simulink model "dcdctest"  (R2023b)
settings: Solver=VariableStepAuto  StartTime=0.0  StopTime=10  RelTol=1e-3
values from neighbouring files (symbols this model uses):
  cell_cap_Ah = 2.2    [find_maximum_ovlp.m]    (also in main.m)
  dst_q_cls = zeros(50, 2)    [main.m]
  dst_trg_soc_av = zeros(50, 1)    [main.m]
  soc = soc_in    [balance_costF.m]    (also in find_maximum_ovlp.m = fix(rand (1, cell_count) * 100); log_clustering.m; main.m = [39    39    20    72    81    92    51    11    60]; plot_final.m)
  src_q_cls = zeros(50, 2)    [main.m]
  src_trg_soc_av = zeros(50, 1)    [main.m]
undefined symbols (not defined in the file or in its folder): Ion, Lithium
libraries: spsIdealSwitchLib x18, spsBatteryLib x12, spsControlledCurrentSourceLib x8, spsVoltageMeasurementLib x8, simulink x4, slpidlib x3, spspowerguiLib x2
(part 1 of 2)
settings Model: NumberOfSteps=100  Creator=10661025  LastModifiedBy=10661025

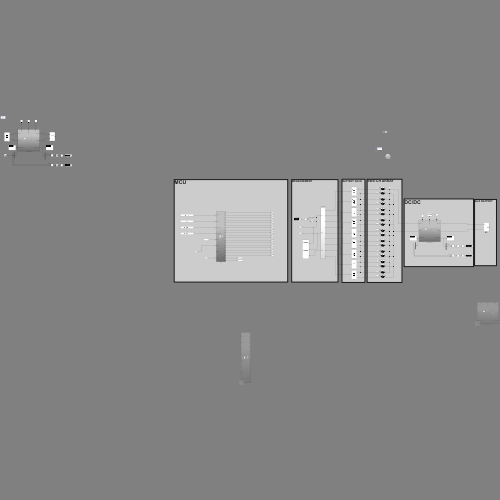
[thumbnail: Simulink's stored preview of the top-level diagram]
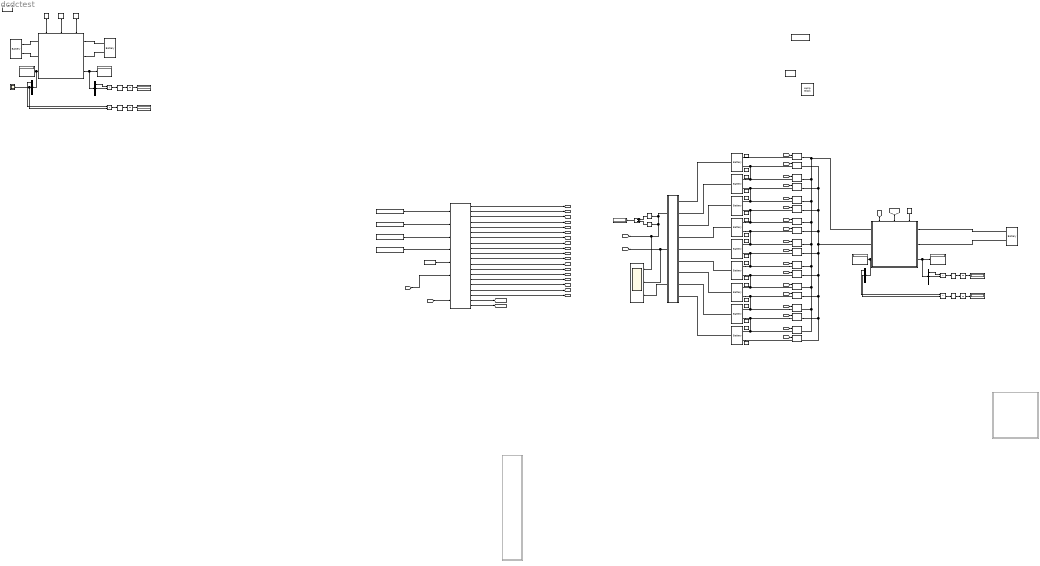
== system dcdctest ==
  note: MCU
  note: DC/DC
  note: MEASUREMENT
  note: BATTERY PACK
  note: SWITCH ARRAY
  note: neg
  note: pos
  note: AUX BATTERY
  Abs{,1..3} (4 alike) : Abs  SaturateOnIntegerOverflow=off
  B1 : spsBatteryLib/Battery  BatType=Lithium-Ion  ShowTempParam=off  ThermalPreset=no  ShowAgeParam=off  NomV=50  NomQ=2.2  SOC=soc(1, 1)  Batt_Tr=30  PresetModel=on  MaxQ=2.2  MinV=37.5  FullV=58.1994  Dis_rate=0.95652  R=0.22727  Normal_OP=1.9896  expZone="[54.0193     0.108087]"  current=[6.5 13 32.5]  Units=Time  Tci=20  NomT=20  T2=-30  MaxQ2=4.8  FullV2=7.1  Normal_OP2=5.655  expZone2="[6.58           1]"  Rca=0.6  ti=2000  Dp=0  Neq0=0  Tsim=1e6  Ta1=25  Qeol=5.4*0.9  Reol=0.013333*1.2  Char_age=[2.3478, 3]  Dis_age=[2.3478, 10]  N1=1500  N2=10500  N3=1000  N4=1400  Ta2=45  N5=950
  B10 : spsBatteryLib/Battery  BatType=Lithium-Ion  ShowTempParam=off  ThermalPreset=no  ShowAgeParam=off  NomV=12  NomQ=60  SOC=soc(1, 1)  Batt_Tr=30  PresetModel=on  MaxQ=60  MinV=9  FullV=13.9678  Dis_rate=26.087  R=0.002  Normal_OP=54.2609  expZone="[12.9646      2.94783]"  current=[6.5 13 32.5]  Units=Time  Tci=20  NomT=20  T2=-30  MaxQ2=4.8  FullV2=7.1  Normal_OP2=5.655  expZone2="[6.58           1]"  Rca=0.6  ti=2000  Dp=0  Neq0=0  Tsim=1e6  Ta1=25  Qeol=5.4*0.9  Reol=0.013333*1.2  Char_age=[2.3478, 3]  Dis_age=[2.3478, 10]  N1=1500  N2=10500  N3=1000  N4=1400  Ta2=45  N5=950
  B11 : spsBatteryLib/Battery  BatType=Lithium-Ion  ShowTempParam=off  ThermalPreset=no  ShowAgeParam=off  NomV=3.7  NomQ=2.2  SOC=soc(1, 8)  Batt_Tr=30  PresetModel=on  MaxQ=2.2  MinV=2.775  FullV=4.3068  Dis_rate=0.95652  R=0.016818  Normal_OP=1.9896  expZone="[3.9974     0.10809]"  current=[6.5 13 32.5]  Units=Time  Tci=20  NomT=20  T2=-30  MaxQ2=4.8  FullV2=7.1  Normal_OP2=5.655  expZone2="[6.58           1]"  Rca=0.6  ti=2000  Dp=0  Neq0=0  Tsim=1e6  Ta1=25  Qeol=5.4*0.9  Reol=0.013333*1.2  Char_age=[2.3478, 3]  Dis_age=[2.3478, 10]  N1=1500  N2=10500  N3=1000  N4=1400  Ta2=45  N5=950
  B12 : spsBatteryLib/Battery  BatType=Lithium-Ion  ShowTempParam=off  ThermalPreset=no  ShowAgeParam=off  NomV=3.7  NomQ=2.2  SOC=soc(1, 9)  Batt_Tr=30  PresetModel=on  MaxQ=2.2  MinV=2.775  FullV=4.3068  Dis_rate=0.95652  R=0.016818  Normal_OP=1.9896  expZone="[3.9974     0.10809]"  current=[6.5 13 32.5]  Units=Time  Tci=20  NomT=20  T2=-30  MaxQ2=4.8  FullV2=7.1  Normal_OP2=5.655  expZone2="[6.58           1]"  Rca=0.6  ti=2000  Dp=0  Neq0=0  Tsim=1e6  Ta1=25  Qeol=5.4*0.9  Reol=0.013333*1.2  Char_age=[2.3478, 3]  Dis_age=[2.3478, 10]  N1=1500  N2=10500  N3=1000  N4=1400  Ta2=45  N5=950
  B2 : spsBatteryLib/Battery  BatType=Lithium-Ion  ShowTempParam=off  ThermalPreset=no  ShowAgeParam=off  NomV=3.7  NomQ=2.2  SOC=soc(1, 1)  Batt_Tr=30  PresetModel=on  MaxQ=2.2  MinV=2.775  FullV=4.3068  Dis_rate=0.95652  R=0.016818  Normal_OP=1.9896  expZone="[3.9974     0.10809]"  current=[6.5 13 32.5]  Units=Time  Tci=20  NomT=20  T2=-30  MaxQ2=4.8  FullV2=7.1  Normal_OP2=5.655  expZone2="[6.58           1]"  Rca=0.6  ti=2000  Dp=0  Neq0=0  Tsim=1e6  Ta1=25  Qeol=5.4*0.9  Reol=0.013333*1.2  Char_age=[2.3478, 3]  Dis_age=[2.3478, 10]  N1=1500  N2=10500  N3=1000  N4=1400  Ta2=45  N5=950
  B3 : spsBatteryLib/Battery  BatType=Lithium-Ion  ShowTempParam=off  ThermalPreset=no  ShowAgeParam=off  NomV=12  NomQ=60  SOC=soc(1, 1)  Batt_Tr=30  PresetModel=on  MaxQ=60  MinV=9  FullV=13.9678  Dis_rate=26.087  R=0.002  Normal_OP=54.2609  expZone="[12.9646      2.94783]"  current=[6.5 13 32.5]  Units=Time  Tci=20  NomT=20  T2=-30  MaxQ2=4.8  FullV2=7.1  Normal_OP2=5.655  expZone2="[6.58           1]"  Rca=0.6  ti=2000  Dp=0  Neq0=0  Tsim=1e6  Ta1=25  Qeol=5.4*0.9  Reol=0.013333*1.2  Char_age=[2.3478, 3]  Dis_age=[2.3478, 10]  N1=1500  N2=10500  N3=1000  N4=1400  Ta2=45  N5=950
  B4 : spsBatteryLib/Battery  BatType=Lithium-Ion  ShowTempParam=off  ThermalPreset=no  ShowAgeParam=off  NomV=3.7  NomQ=2.2  SOC=soc(1, 2)  Batt_Tr=30  PresetModel=on  MaxQ=2.2  MinV=2.775  FullV=4.3068  Dis_rate=0.95652  R=0.016818  Normal_OP=1.9896  expZone="[3.9974     0.10809]"  current=[6.5 13 32.5]  Units=Time  Tci=20  NomT=20  T2=-30  MaxQ2=4.8  FullV2=7.1  Normal_OP2=5.655  expZone2="[6.58           1]"  Rca=0.6  ti=2000  Dp=0  Neq0=0  Tsim=1e6  Ta1=25  Qeol=5.4*0.9  Reol=0.013333*1.2  Char_age=[2.3478, 3]  Dis_age=[2.3478, 10]  N1=1500  N2=10500  N3=1000  N4=1400  Ta2=45  N5=950
  B5 : spsBatteryLib/Battery  BatType=Lithium-Ion  ShowTempParam=off  ThermalPreset=no  ShowAgeParam=off  NomV=3.7  NomQ=2.2  SOC=soc(1, 3)  Batt_Tr=30  PresetModel=on  MaxQ=2.2  MinV=2.775  FullV=4.3068  Dis_rate=0.95652  R=0.016818  Normal_OP=1.9896  expZone="[3.9974     0.10809]"  current=[6.5 13 32.5]  Units=Time  Tci=20  NomT=20  T2=-30  MaxQ2=4.8  FullV2=7.1  Normal_OP2=5.655  expZone2="[6.58           1]"  Rca=0.6  ti=2000  Dp=0  Neq0=0  Tsim=1e6  Ta1=25  Qeol=5.4*0.9  Reol=0.013333*1.2  Char_age=[2.3478, 3]  Dis_age=[2.3478, 10]  N1=1500  N2=10500  N3=1000  N4=1400  Ta2=45  N5=950
  B6 : spsBatteryLib/Battery  BatType=Lithium-Ion  ShowTempParam=off  ThermalPreset=no  ShowAgeParam=off  NomV=3.7  NomQ=2.2  SOC=soc(1, 4)  Batt_Tr=30  PresetModel=on  MaxQ=2.2  MinV=2.775  FullV=4.3068  Dis_rate=0.95652  R=0.016818  Normal_OP=1.9896  expZone="[3.9974     0.10809]"  current=[6.5 13 32.5]  Units=Time  Tci=20  NomT=20  T2=-30  MaxQ2=4.8  FullV2=7.1  Normal_OP2=5.655  expZone2="[6.58           1]"  Rca=0.6  ti=2000  Dp=0  Neq0=0  Tsim=1e6  Ta1=25  Qeol=5.4*0.9  Reol=0.013333*1.2  Char_age=[2.3478, 3]  Dis_age=[2.3478, 10]  N1=1500  N2=10500  N3=1000  N4=1400  Ta2=45  N5=950
  B7 : spsBatteryLib/Battery  BatType=Lithium-Ion  ShowTempParam=off  ThermalPreset=no  ShowAgeParam=off  NomV=3.7  NomQ=2.2  SOC=soc(1, 5)  Batt_Tr=30  PresetModel=on  MaxQ=2.2  MinV=2.775  FullV=4.3068  Dis_rate=0.95652  R=0.016818  Normal_OP=1.9896  expZone="[3.9974     0.10809]"  current=[6.5 13 32.5]  Units=Time  Tci=20  NomT=20  T2=-30  MaxQ2=4.8  FullV2=7.1  Normal_OP2=5.655  expZone2="[6.58           1]"  Rca=0.6  ti=2000  Dp=0  Neq0=0  Tsim=1e6  Ta1=25  Qeol=5.4*0.9  Reol=0.013333*1.2  Char_age=[2.3478, 3]  Dis_age=[2.3478, 10]  N1=1500  N2=10500  N3=1000  N4=1400  Ta2=45  N5=950
  B8 : spsBatteryLib/Battery  BatType=Lithium-Ion  ShowTempParam=off  ThermalPreset=no  ShowAgeParam=off  NomV=3.7  NomQ=2.2  SOC=soc(1, 6)  Batt_Tr=30  PresetModel=on  MaxQ=2.2  MinV=2.775  FullV=4.3068  Dis_rate=0.95652  R=0.016818  Normal_OP=1.9896  expZone="[3.9974     0.10809]"  current=[6.5 13 32.5]  Units=Time  Tci=20  NomT=20  T2=-30  MaxQ2=4.8  FullV2=7.1  Normal_OP2=5.655  expZone2="[6.58           1]"  Rca=0.6  ti=2000  Dp=0  Neq0=0  Tsim=1e6  Ta1=25  Qeol=5.4*0.9  Reol=0.013333*1.2  Char_age=[2.3478, 3]  Dis_age=[2.3478, 10]  N1=1500  N2=10500  N3=1000  N4=1400  Ta2=45  N5=950
  B9 : spsBatteryLib/Battery  BatType=Lithium-Ion  ShowTempParam=off  ThermalPreset=no  ShowAgeParam=off  NomV=3.7  NomQ=2.2  SOC=soc(1, 7)  Batt_Tr=30  PresetModel=on  MaxQ=2.2  MinV=2.775  FullV=4.3068  Dis_rate=0.95652  R=0.016818  Normal_OP=1.9896  expZone="[3.9974     0.10809]"  current=[6.5 13 32.5]  Units=Time  Tci=20  NomT=20  T2=-30  MaxQ2=4.8  FullV2=7.1  Normal_OP2=5.655  expZone2="[6.58           1]"  Rca=0.6  ti=2000  Dp=0  Neq0=0  Tsim=1e6  Ta1=25  Qeol=5.4*0.9  Reol=0.013333*1.2  Char_age=[2.3478, 3]  Dis_age=[2.3478, 10]  N1=1500  N2=10500  N3=1000  N4=1400  Ta2=45  N5=950
  Constant : Constant  Value=src_q_cls
  Constant1 : Constant
  Constant2 : Constant  Value=dst_q_cls
  Constant3 : Constant  Value=2
  Constant4 : Constant  Value=src_trg_soc_av
  Constant5 : Constant  Value=dst_trg_soc_av
  Constant6 : Constant  Value=cell_cap_Ah
  DC-DC converter : Subsystem
      settings: PortSchema="{\"entries\":[{\"content\":{\"sides\":[{\"content\":{\"connectorIds\":[\"LConn1\",\"LConn2\",\"Out2\"]},\"type\":\"ConnectorPlacement.EquallySpacedRectSide\",\"uuid\":\"b8e9ea21-fc6f-4abe-9815-7c96c8754cc1\"},{\"content\":{\"connectorIds\":[\"RConn1\",\"RConn2\",\"Out1\"],\"side\":\"RIGHT\"},\"type\":\"ConnectorPlacement.EquallySpacedRectSide\",\"uuid\":\"546bb611-6f28-45af-a15a-a960a3093258\"},{\"content\":{\"connectorIds\":[\"In1\",\"In2\",\"In3\"],\"side\":\"TOP\"},\"type\":\"ConnectorPlacement.EquallySpacedRectSide\",\"uuid\":\"f1a81754-76ae-41da-bcef-17d54c1fc977\"}]},\"type\":\"ConnectorPlacement.EquallySpacedConnector\",\"uuid\":\"f395fac5-4dd1-431a-bb8e-7682cfb9cc98\"}],\"packageUris\":[\"http://schema.mathworks.com/mf0/Connector/R2020b\"],\"version\":\"1.0\"}"
  DC-DC converter1 : Subsystem  Commented=on
      settings: PortSchema="{\"entries\":[{\"content\":{\"sides\":[{\"content\":{\"connectorIds\":[\"LConn1\",\"LConn2\",\"Out2\"]},\"type\":\"ConnectorPlacement.EquallySpacedRectSide\",\"uuid\":\"b8e9ea21-fc6f-4abe-9815-7c96c8754cc1\"},{\"content\":{\"connectorIds\":[\"RConn1\",\"RConn2\",\"Out1\"],\"side\":\"RIGHT\"},\"type\":\"ConnectorPlacement.EquallySpacedRectSide\",\"uuid\":\"546bb611-6f28-45af-a15a-a960a3093258\"},{\"content\":{\"connectorIds\":[\"In1\",\"In2\",\"In3\"],\"side\":\"TOP\"},\"type\":\"ConnectorPlacement.EquallySpacedRectSide\",\"uuid\":\"f1a81754-76ae-41da-bcef-17d54c1fc977\"}]},\"type\":\"ConnectorPlacement.EquallySpacedConnector\",\"uuid\":\"f395fac5-4dd1-431a-bb8e-7682cfb9cc98\"}],\"packageUris\":[\"http://schema.mathworks.com/mf0/Connector/R2020b\"],\"version\":\"1.0\"}"
  DC-DC converter2 : Subsystem
      settings: PortSchema="{\"entries\":[{\"content\":{\"sides\":[{\"content\":{\"connectorIds\":[\"LConn1\",\"LConn2\",\"Out2\"]},\"type\":\"ConnectorPlacement.EquallySpacedRectSide\",\"uuid\":\"b8e9ea21-fc6f-4abe-9815-7c96c8754cc1\"},{\"content\":{\"connectorIds\":[\"RConn1\",\"RConn2\",\"Out1\"],\"side\":\"RIGHT\"},\"type\":\"ConnectorPlacement.EquallySpacedRectSide\",\"uuid\":\"546bb611-6f28-45af-a15a-a960a3093258\"},{\"content\":{\"connectorIds\":[\"In1\",\"In2\",\"In3\"],\"side\":\"TOP\"},\"type\":\"ConnectorPlacement.EquallySpacedRectSide\",\"uuid\":\"f1a81754-76ae-41da-bcef-17d54c1fc977\"}]},\"type\":\"ConnectorPlacement.EquallySpacedConnector\",\"uuid\":\"f395fac5-4dd1-431a-bb8e-7682cfb9cc98\"}],\"packageUris\":[\"http://schema.mathworks.com/mf0/Connector/R2020b\"],\"version\":\"1.0\"}"
  Demux{,1..3} (4 alike) : Demux  Outputs=3
  Display{,1..7} (8 alike) : Display
  Ideal Switch{,1..17} (18 alike) : spsIdealSwitchLib/Ideal Switch  Ron=0.001  Lon=0  IC=0  Rs=1e5  Cs=inf  Measurements=on
  Integrator{,1..3} (4 alike) : Integrator
  Lamp{,1..18} (19 alike) : LampBlock  LabelPosition=Hide
  MinMax : MinMax  Function=max
  MinMax1 : MinMax
  Product{,1..3} (4 alike) : Product
  Scope : Scope
  Scope1 : Scope  NumInputPorts=3
  Slider Switch : SliderSwitchBlock
      settings: Values={{'Off', 'On'}, [0 1]}
  Subtract : Sum  Inputs=+-
  e : Constant
  e1 : Constant
  inconsistency : Display
  mcu : Subsystem  Commented=on
  mcu1 : Subsystem
  measurement : Subsystem
  powergui : spspowerguiLib/powergui  Priority=1  SimulationMode=Discrete  SampleTime=1E-3  frequency=60  Iterations=50  frequencyindice=0  Pbase=100e6  ErrMax=1e-4  UnitsV=kV  UnitsW=MW  buscounter=0  FunctionMessages=off  echomessages=off  EnableUseOfTLC=off  CurrentSourceSwitches=off  DisableSnubberDevices=off  DisableRonSwitches=off  DisableVfSwitches=off  DisplayEquations=off  AutomaticDiscreteSolvers=off  SolverType=Tustin/Backward Euler (TBE)  Interpol=off  ExternalGateDelay=off  methode=on  Ts=1000  x0status=blocks  SPID=off  SwTol=0  HookPort=off  NonlinearTolerance=1e-4  nMaxIteration=10  ContinueOnMaxIteration=off  RestoreLinks=warning  ResistiveCurrentMeasurement=off  Frange=[0:2:500]  Ylog=off  Xlog=on  ShowGrid=off  save=off  variable=ZData  structure=0  ZoomFFT=off  StartTime=0.0  cycles=1  DisplayStyle=1  fundamental=60  FreqAxis=off  MaxFrequency=1000  frequencyindicesteady=1  RmsSteady=1  display=off
  powergui1 : spspowerguiLib/powergui  Priority=1  SimulationMode=Discrete  SampleTime=1E-3  frequency=60  Iterations=50  frequencyindice=0  Pbase=100e6  ErrMax=1e-4  UnitsV=kV  UnitsW=MW  buscounter=0  FunctionMessages=off  echomessages=off  EnableUseOfTLC=off  CurrentSourceSwitches=off  DisableSnubberDevices=off  DisableRonSwitches=off  DisableVfSwitches=off  DisplayEquations=off  AutomaticDiscreteSolvers=off  SolverType=Tustin/Backward Euler (TBE)  Interpol=off  ExternalGateDelay=off  methode=on  Ts=1000  x0status=blocks  SPID=off  SwTol=0  HookPort=off  NonlinearTolerance=1e-4  nMaxIteration=10  ContinueOnMaxIteration=off  RestoreLinks=warning  ResistiveCurrentMeasurement=off  Frange=[0:2:500]  Ylog=off  Xlog=on  ShowGrid=off  save=off  variable=ZData  structure=0  ZoomFFT=off  StartTime=0.0  cycles=1  DisplayStyle=1  fundamental=60  FreqAxis=off  MaxFrequency=1000  frequencyindicesteady=1  RmsSteady=1  display=off
  wires:
  Abs1/1 -> Integrator1/1
  Demux2/1 -> Product/1  "V_cap"
  DC-DC converter/1(Outport) -> Display2/1, Demux2/1
  DC-DC converter/2(Outport1) -> Demux/1, Display3/1
  Abs/1 -> Integrator/1
  Constant1/1 -> DC-DC converter/1(direction)
  Demux2/2 -> Product/2  "Iout"
  e/1 -> DC-DC converter/3(enable)
  Demux/2 -> Scope/1, Product1/2  "Iout"
  Demux/1 -> Product1/1  "V_cap"
  Product/1 -> Abs/1
  Integrator1/1 -> Display4/1
  Product1/1 -> Abs1/1
  Integrator/1 -> Display/1
  Constant3/1 -> DC-DC converter/2(current_desired)
  Abs3/1 -> Integrator3/1
  [eq_current] -> DC-DC converter2/2(current_desired)
  [dir] -> DC-DC converter2/1(direction)
  DC-DC converter2/2(Outport1) -> Demux1/1, Display6/1
  DC-DC converter2/1(Outport) -> Display5/1, Demux3/1
  e1/1 -> DC-DC converter2/3(enable)
  measurement/2(current) -> Scope1/2, [current]
  Demux3/1 -> Product2/1  "V_cap"
  Abs2/1 -> Integrator2/1
  [g2p] -> Ideal Switch10/1
  B7/1 -> measurement/5(In5)
  B6/1 -> measurement/4(In4)
  [g4p] -> Ideal Switch4/1
  [g9p] -> Ideal Switch17/1
  B9/1 -> measurement/7(In7)
  B8/1 -> measurement/6(In6)
  Demux3/2 -> Product2/2  "Iout"
  MinMax/1 -> Subtract/1
  measurement/3(voltage) -> Scope1/3
  [g9n] -> Ideal Switch15/1
  B4/1 -> measurement/2(In2)
  [g7n] -> Ideal Switch9/1
  [g7p] -> Ideal Switch13/1
  [g8p] -> Ideal Switch14/1
  [g3p] -> Ideal Switch3/1
  [g5p] -> Ideal Switch7/1
  [g5n] -> Ideal Switch5/1
  Demux1/2 -> Product3/2  "Iout"
  Product2/1 -> Abs2/1
  Demux1/1 -> Product3/1  "V_cap"
  B12/1 -> measurement/9(In9)
  [g4n] -> Ideal Switch6/1
  Product3/1 -> Abs3/1
  [g1n] -> Ideal Switch/1
  MinMax1/1 -> Subtract/2
  [g6n] -> Ideal Switch12/1
  [SOC] -> mcu1/6(CAP_Ah)
  [g6p] -> Ideal Switch8/1
  mcu1/19(eq_current) -> [eq_current]
  Subtract/1 -> inconsistency/1
  mcu1/20(dir) -> [dir]
  mcu1/18(g9n) -> [g9n]
  Integrator2/1 -> Display1/1
  B2/1 -> measurement/1(In1)
  mcu1/14(g5n) -> [g5n]
  mcu1/16(g7n) -> [g7n]
  mcu1/17(g8n) -> [g8n]
  mcu1/3(g3p) -> [g3p]
  mcu1/5(g5p) -> [g5p]
  Constant5/1 -> mcu1/4(dst_trg_soc_av)
  B5/1 -> measurement/3(In3)
  B11/1 -> measurement/8(In8)
  mcu1/11(g2n) -> [g2n]
  mcu1/13(g4n) -> [g4n]
  [g8n] -> Ideal Switch16/1
  mcu1/7(g7p) -> [g7p]
  mcu1/9(g9p) -> [g9p]
  Constant4/1 -> mcu1/3(src_trg_soc_av)
  mcu1/15(g6n) -> [g6n]
  mcu1/12(g3n) -> [g3n]
  Constant2/1 -> mcu1/2(dst_q_cls)
  measurement/1(SOC) -> MinMax/1, MinMax1/1, Scope1/1, [SOC]
  Integrator3/1 -> Display7/1
  mcu1/4(g4p) -> [g4p]
  mcu1/6(g6p) -> [g6p]
  mcu1/10(g1n) -> [g1n]
  mcu1/1(g1p) -> [g1p]
  [g1p] -> Ideal Switch1/1
  mcu1/2(g2p) -> [g2p]
  Constant6/1 -> mcu1/5(SOC)
  [g3n] -> Ideal Switch11/1
  Constant/1 -> mcu1/1(src_q_cls)
  [current] -> mcu1/8(I_meas)
  [g2n] -> Ideal Switch2/1
  mcu1/8(g8p) -> [g8p]
  connections:
  DC-DC converter/RConn2 -- B10/LConn2
  DC-DC converter/RConn1 -- B10/LConn1
  B1/LConn1 -- DC-DC converter/LConn1
  B1/LConn2 -- DC-DC converter/LConn2
  Ideal Switch12/RConn1 -- DC-DC converter2/LConn2 -- Ideal Switch/RConn1 -- Ideal Switch2/RConn1 -- Ideal Switch11/RConn1 -- Ideal Switch6/RConn1 -- Ideal Switch5/RConn1 -- Ideal Switch16/RConn1 -- Ideal Switch15/RConn1 -- Ideal Switch9/RConn1
  Ideal Switch16/LConn1 -- B11/LConn2 -- Ideal Switch17/LConn1 -- B12/LConn1
  Ideal Switch8/LConn1 -- B8/LConn1 -- Ideal Switch5/LConn1 -- B7/LConn2
  B2/LConn2 -- Ideal Switch/LConn1 -- Ideal Switch10/LConn1 -- B4/LConn1
  B7/LConn1 -- B6/LConn2 -- Ideal Switch6/LConn1 -- Ideal Switch7/LConn1
  B5/LConn2 -- B6/LConn1 -- Ideal Switch4/LConn1 -- Ideal Switch11/LConn1
  Ideal Switch13/RConn1 -- DC-DC converter2/LConn1 -- Ideal Switch1/RConn1 -- Ideal Switch10/RConn1 -- Ideal Switch3/RConn1 -- Ideal Switch4/RConn1 -- Ideal Switch7/RConn1 -- Ideal Switch8/RConn1 -- Ideal Switch17/RConn1 -- Ideal Switch14/RConn1
  B5/LConn1 -- Ideal Switch2/LConn1 -- B4/LConn2 -- Ideal Switch3/LConn1
  B9/LConn1 -- B8/LConn2 -- Ideal Switch12/LConn1 -- Ideal Switch13/LConn1
  Ideal Switch14/LConn1 -- B11/LConn1 -- B9/LConn2 -- Ideal Switch9/LConn1
  DC-DC converter2/RConn2 -- B3/LConn2
  DC-DC converter2/RConn1 -- B3/LConn1
  Ideal Switch1/LConn1 -- B2/LConn1
  B12/LConn2 -- Ideal Switch15/LConn1

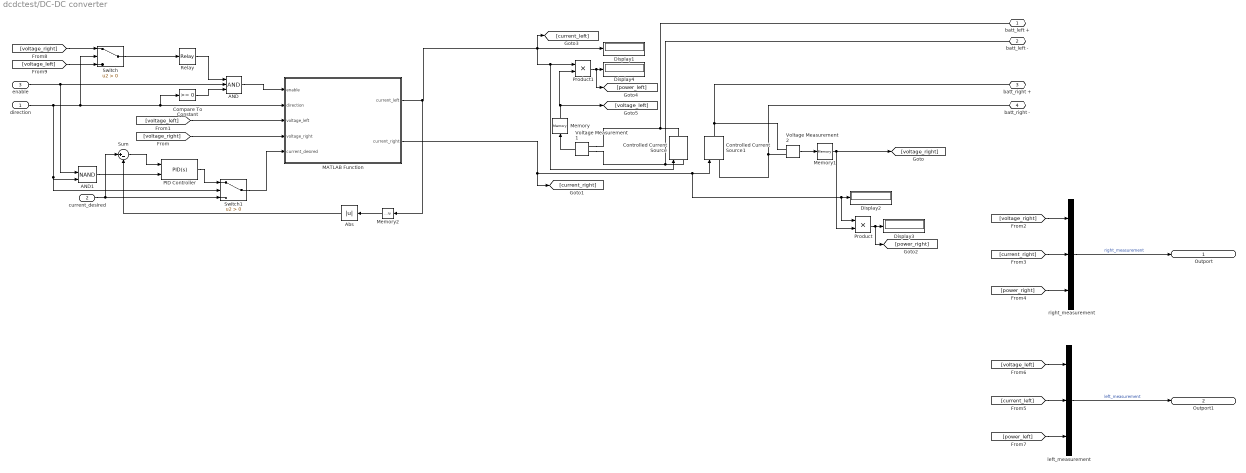
== system dcdctest/DC-DC converter ==
  direction : Inport
  current_desired : Inport  Port=2
  enable : Inport  Port=3
  AND : Logic  Inputs=3  IconShape=distinctive  AllPortsSameDT=off  OutDataTypeStr=boolean
  AND1 : Logic  Operator=NAND  IconShape=distinctive  AllPortsSameDT=off  OutDataTypeStr=boolean
  Abs : Abs  SaturateOnIntegerOverflow=off
  Compare To Constant : simulink/Logic and Bit Operations/Compare To Constant  relop=>=  const=0  OutDataTypeStr=boolean
  Controlled Current Source : spsControlledCurrentSourceLib/Controlled Current Source  Initialize=on  Source_Type=DC  Amplitude=0  Phase=0  Frequency=0  Measurements=None
  Controlled Current Source1 : spsControlledCurrentSourceLib/Controlled Current Source  Initialize=on  Source_Type=AC  Amplitude=0  Phase=0  Frequency=0  Measurements=None
  Display{1..4} (4 alike) : Display
  MATLAB Function : MATLAB Function  TreatAsAtomicUnit=on
  Memory : Memory
  Memory1 : Memory
  Memory2 : Memory
  PID Controller : slpidlib/PID Controller  Controller=PID  Form=Parallel  TimeDomain=Continuous-time  UseExternalTs=off  SampleTime=-1  IntegratorMethod=Forward Euler  FilterMethod=Forward Euler  ControllerParametersSource=internal  P=0.01  I=2  UseKiTs=off  D=0  N=100  UseFilter=on  TunerSelectOption=Transfer Function Based (PID Tuner App)  InitialConditionSource=internal  InitialConditionForIntegrator=0  InitialConditionForFilter=0  DifferentiatorICPrevScaledInput=0  ExternalReset=level  TrackingMode=off  Kt=1  LimitOutput=on  SatLimitsSource=internal  UpperSaturationLimit=2  LowerSaturationLimit=0  LinearizeAsGain=on  AntiWindupMode=none  Kb=1  LimitIntegrator=off  UpperIntegratorSaturationLimit=inf  LowerIntegratorSaturationLimit=-inf  POutMin=[]  POutMax=[]  IOutMin=[]  IOutMax=[]  DOutMin=[]  DOutMax=[]  NOutMin=[]  NOutMax=[]  SumOutMin=[]  SumOutMax=[]  SaturationOutMin=[]  SaturationOutMax=[]  PParamMin=[]  PParamMax=[]  IParamMin=[]  IParamMax=[]  DParamMin=[]  DParamMax=[]  NParamMin=[]  NParamMax=[]  KbParamMin=[]  KbParamMax=[]  KtParamMin=[]  KtParamMax=[]  KbOutMin=[]  KbOutMax=[]  KtOutMin=[]  KtOutMax=[]  IntegratorOutMin=[]  IntegratorOutMax=[]  FilterOutMin=[]  FilterOutMax=[]  SumI1OutMin=[]  SumI1OutMax=[]  SumI2OutMin=[]  SumI2OutMax=[]  SumI3OutMin=[]  SumI3OutMax=[]  SumI4OutMin=[]  SumI4OutMax=[]  SumDOutMin=[]  SumDOutMax=[]  DifferentiatorOutMin=[]  DifferentiatorOutMax=[]  FilterDiffOutCoefMin=[]  FilterDiffOutCoefMax=[]  ReciprocalOutMin=[]  ReciprocalOutMax=[]  SumDenOutMin=[]  SumDenOutMax=[]  SumNumOutMin=[]  SumNumOutMax=[]  DivideOutMin=[]  DivideOutMax=[]  UdiffTsProdOutMin=[]  UdiffTsProdOutMax=[]  NTsProdOutMin=[]  NTsProdOutMax=[]  UintegralTsProdOutMin=[]  UintegralTsProdOutMax=[]  UngainTsProdOutMin=[]  UngainTsProdOutMax=[]  ClampingZeroOutDataTypeStr=Inherit: Inherit via back propagation  ClampingZeroOutMin=[]  ClampingZeroOutMax=[]  FilterDenConstantOutDataTypeStr=Inherit: Inherit via back propagation  FilterDenConstantOutMin=[]  FilterDenConstantOutMax=[]  PCopyOutDataTypeStr=Inherit: Inherit via back propagation  PCopyOutMin=[]  PCopyOutMax=[]  NCopyOutDataTypeStr=Inherit: Inherit via back propagation  NCopyOutMin=[]  NCopyOutMax=[]  IntegratorContinuousStateAttributes=''  IntegratorStateMustResolveToSignalObject=off  IntegratorRTWStateStorageClass=Auto  FilterContinuousStateAttributes=''  FilterStateMustResolveToSignalObject=off  FilterRTWStateStorageClass=Auto  ParallelPVariant=InternalParameters  IdealPVariant=Disabled  IVariant=InternalParameters  DVariant=InternalParameters  IntegratorVariant=Continuous  SatVariant=Enabled  AWVariant=Passthrough  PCopyVariant=Disabled  TRVariant=Disabled  FdbkBlocksVariant=Forward  IdealPFdbkVariant=Disabled  SatFdbkVariant=Disabled  DerivativeFilterVariant=ContFilter  NVariant=InternalParameters  NCopyVariant=Disabled  FilterICVariant=InternalICsFilter  IntegratorICVariant=InternalICs  ExternalResetVariant=ExternalReset  TRSumVariant=Passthrough  SumFdbkVariant=Disabled  SumVariant=Sum_PID  TsampFilterVariant=InternalTs  TsampNgainVariant=Passthrough  TsampIntegralVariant=Disabled_SignalSpec  ExternalSaturationOutDataTypeStr=Inherit: Same as second input
  Product : Product
  Product1 : Product
  Relay : Relay  OnSwitchValue=3.5  OffSwitchValue=2
  Sum : Sum  Inputs=|+-
  Switch : Switch  Criteria=u2 > Threshold  SaturateOnIntegerOverflow=off  InputSameDT=off
  Switch1 : Switch  Criteria=u2 > Threshold  SaturateOnIntegerOverflow=off  InputSameDT=off
  Voltage Measurement1 : spsVoltageMeasurementLib/Voltage Measurement  PhasorSimulation=off  OutputType=Complex  PSBequivalent=0
  Voltage Measurement2 : spsVoltageMeasurementLib/Voltage Measurement  PhasorSimulation=off  OutputType=Complex  PSBequivalent=0
  left_measurement : Mux  Inputs=3
  right_measurement : Mux  Inputs=3
  batt_left + : PMIOPort  Side=Left
  batt_left - : PMIOPort  Port=2  Side=Left
  batt_right + : PMIOPort  Port=3  Side=Right
  batt_right - : PMIOPort  Port=4  Side=Right
  Outport : Outport
  Outport1 : Outport  Port=2
  wires:
  MATLAB Function/1(current_left) -> Memory2/1, Controlled Current Source/1, Product1/1, [current_left], Display1/1
  enable/1 -> AND1/1, AND/2
  Voltage Measurement2/1 -> Memory1/1
  direction/1 -> Compare To Constant/1, MATLAB Function/2(direction), Switch/2, AND1/2, Switch1/2
  [voltage_right] -> MATLAB Function/4(voltage_right)
  [voltage_left] -> MATLAB Function/3(voltage_left)
  Product/1 -> [power_right], Display3/1
  Product1/1 -> [power_left], Display4/1
  current_desired/1 -> Sum/1, Switch1/3
  [voltage_right] -> right_measurement/1
  [current_right] -> right_measurement/2
  [power_right] -> right_measurement/3
  [power_left] -> left_measurement/3
  [current_left] -> left_measurement/2
  [voltage_left] -> left_measurement/1
  right_measurement/1 -> Outport/1  "right_measurement"
  left_measurement/1 -> Outport1/1  "left_measurement"
  Voltage Measurement1/1 -> Memory/1
  Relay/1 -> AND/1
  AND/1 -> MATLAB Function/1(enable)
  Switch/1 -> Relay/1
  [voltage_left] -> Switch/3
  [voltage_right] -> Switch/1
  Memory/1 -> Product1/2, [voltage_left]
  Memory1/1 -> [voltage_right], Product/2
  Compare To Constant/1 -> AND/3
  Sum/1 -> PID Controller/1
  PID Controller/1 -> Switch1/1
  Switch1/1 -> MATLAB Function/5(current_desired)
  AND1/1 -> PID Controller/2
  Memory2/1 -> Abs/1
  MATLAB Function/2(current_right) -> [current_right], Product/1, Display2/1, Controlled Current Source1/1
  Abs/1 -> Sum/2
  connections:
  Voltage Measurement1/LConn1 -- batt_left +/RConn1 -- Controlled Current Source/RConn1
  Controlled Current Source1/RConn1 -- batt_right +/RConn1 -- Voltage Measurement2/LConn1
  Voltage Measurement2/LConn2 -- Controlled Current Source1/LConn1 -- batt_right -/RConn1
  Voltage Measurement1/LConn2 -- batt_left -/RConn1 -- Controlled Current Source/LConn1

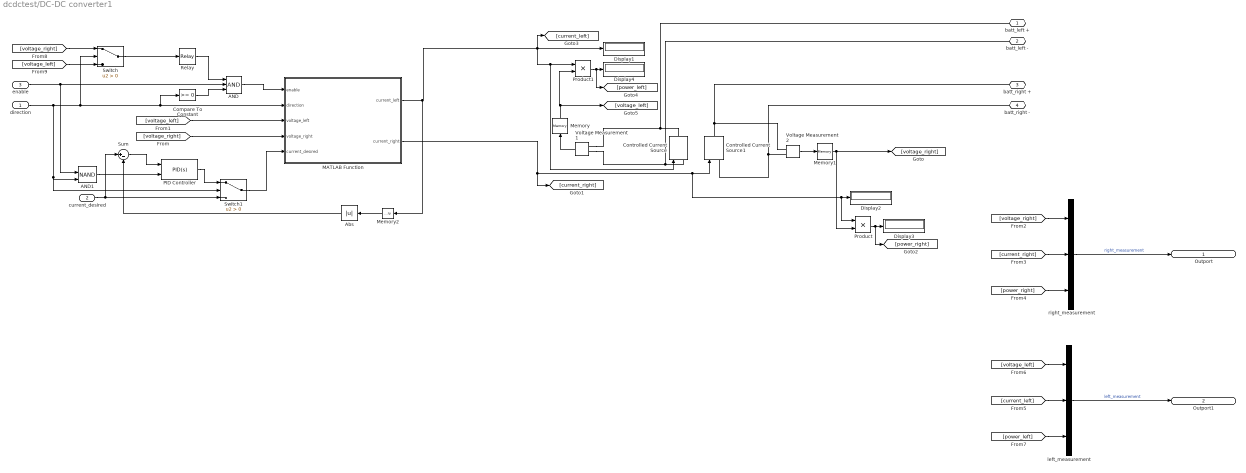
== system dcdctest/DC-DC converter1 ==
  direction : Inport
  current_desired : Inport  Port=2
  enable : Inport  Port=3
  AND : Logic  Inputs=3  IconShape=distinctive  AllPortsSameDT=off  OutDataTypeStr=boolean
  AND1 : Logic  Operator=NAND  IconShape=distinctive  AllPortsSameDT=off  OutDataTypeStr=boolean
  Abs : Abs  SaturateOnIntegerOverflow=off
  Compare To Constant : simulink/Logic and Bit Operations/Compare To Constant  relop=>=  const=0  OutDataTypeStr=boolean
  Controlled Current Source : spsControlledCurrentSourceLib/Controlled Current Source  Initialize=on  Source_Type=DC  Amplitude=0  Phase=0  Frequency=0  Measurements=None
  Controlled Current Source1 : spsControlledCurrentSourceLib/Controlled Current Source  Initialize=on  Source_Type=AC  Amplitude=0  Phase=0  Frequency=0  Measurements=None
  Display{1..4} (4 alike) : Display
  MATLAB Function : MATLAB Function  TreatAsAtomicUnit=on
  Memory : Memory
  Memory1 : Memory
  Memory2 : Memory
  PID Controller : slpidlib/PID Controller  Controller=PID  Form=Parallel  TimeDomain=Continuous-time  UseExternalTs=off  SampleTime=-1  IntegratorMethod=Forward Euler  FilterMethod=Forward Euler  ControllerParametersSource=internal  P=0.01  I=2  UseKiTs=off  D=0  N=100  UseFilter=on  TunerSelectOption=Transfer Function Based (PID Tuner App)  InitialConditionSource=internal  InitialConditionForIntegrator=0  InitialConditionForFilter=0  DifferentiatorICPrevScaledInput=0  ExternalReset=level  TrackingMode=off  Kt=1  LimitOutput=on  SatLimitsSource=internal  UpperSaturationLimit=2  LowerSaturationLimit=0  LinearizeAsGain=on  AntiWindupMode=none  Kb=1  LimitIntegrator=off  UpperIntegratorSaturationLimit=inf  LowerIntegratorSaturationLimit=-inf  POutMin=[]  POutMax=[]  IOutMin=[]  IOutMax=[]  DOutMin=[]  DOutMax=[]  NOutMin=[]  NOutMax=[]  SumOutMin=[]  SumOutMax=[]  SaturationOutMin=[]  SaturationOutMax=[]  PParamMin=[]  PParamMax=[]  IParamMin=[]  IParamMax=[]  DParamMin=[]  DParamMax=[]  NParamMin=[]  NParamMax=[]  KbParamMin=[]  KbParamMax=[]  KtParamMin=[]  KtParamMax=[]  KbOutMin=[]  KbOutMax=[]  KtOutMin=[]  KtOutMax=[]  IntegratorOutMin=[]  IntegratorOutMax=[]  FilterOutMin=[]  FilterOutMax=[]  SumI1OutMin=[]  SumI1OutMax=[]  SumI2OutMin=[]  SumI2OutMax=[]  SumI3OutMin=[]  SumI3OutMax=[]  SumI4OutMin=[]  SumI4OutMax=[]  SumDOutMin=[]  SumDOutMax=[]  DifferentiatorOutMin=[]  DifferentiatorOutMax=[]  FilterDiffOutCoefMin=[]  FilterDiffOutCoefMax=[]  ReciprocalOutMin=[]  ReciprocalOutMax=[]  SumDenOutMin=[]  SumDenOutMax=[]  SumNumOutMin=[]  SumNumOutMax=[]  DivideOutMin=[]  DivideOutMax=[]  UdiffTsProdOutMin=[]  UdiffTsProdOutMax=[]  NTsProdOutMin=[]  NTsProdOutMax=[]  UintegralTsProdOutMin=[]  UintegralTsProdOutMax=[]  UngainTsProdOutMin=[]  UngainTsProdOutMax=[]  ClampingZeroOutDataTypeStr=Inherit: Inherit via back propagation  ClampingZeroOutMin=[]  ClampingZeroOutMax=[]  FilterDenConstantOutDataTypeStr=Inherit: Inherit via back propagation  FilterDenConstantOutMin=[]  FilterDenConstantOutMax=[]  PCopyOutDataTypeStr=Inherit: Inherit via back propagation  PCopyOutMin=[]  PCopyOutMax=[]  NCopyOutDataTypeStr=Inherit: Inherit via back propagation  NCopyOutMin=[]  NCopyOutMax=[]  IntegratorContinuousStateAttributes=''  IntegratorStateMustResolveToSignalObject=off  IntegratorRTWStateStorageClass=Auto  FilterContinuousStateAttributes=''  FilterStateMustResolveToSignalObject=off  FilterRTWStateStorageClass=Auto  ParallelPVariant=InternalParameters  IdealPVariant=Disabled  IVariant=InternalParameters  DVariant=InternalParameters  IntegratorVariant=Continuous  SatVariant=Enabled  AWVariant=Passthrough  PCopyVariant=Disabled  TRVariant=Disabled  FdbkBlocksVariant=Forward  IdealPFdbkVariant=Disabled  SatFdbkVariant=Disabled  DerivativeFilterVariant=ContFilter  NVariant=InternalParameters  NCopyVariant=Disabled  FilterICVariant=InternalICsFilter  IntegratorICVariant=InternalICs  ExternalResetVariant=ExternalReset  TRSumVariant=Passthrough  SumFdbkVariant=Disabled  SumVariant=Sum_PID  TsampFilterVariant=InternalTs  TsampNgainVariant=Passthrough  TsampIntegralVariant=Disabled_SignalSpec  ExternalSaturationOutDataTypeStr=Inherit: Same as second input
  Product : Product
  Product1 : Product
  Relay : Relay  OnSwitchValue=3.5  OffSwitchValue=2
  Sum : Sum  Inputs=|+-
  Switch : Switch  Criteria=u2 > Threshold  SaturateOnIntegerOverflow=off  InputSameDT=off
  Switch1 : Switch  Criteria=u2 > Threshold  SaturateOnIntegerOverflow=off  InputSameDT=off
  Voltage Measurement1 : spsVoltageMeasurementLib/Voltage Measurement  PhasorSimulation=off  OutputType=Complex  PSBequivalent=0
  Voltage Measurement2 : spsVoltageMeasurementLib/Voltage Measurement  PhasorSimulation=off  OutputType=Complex  PSBequivalent=0
  left_measurement : Mux  Inputs=3
  right_measurement : Mux  Inputs=3
  batt_left + : PMIOPort  Side=Left
  batt_left - : PMIOPort  Port=2  Side=Left
  batt_right + : PMIOPort  Port=3  Side=Right
  batt_right - : PMIOPort  Port=4  Side=Right
  Outport : Outport
  Outport1 : Outport  Port=2
  wires:
  MATLAB Function/1(current_left) -> Memory2/1, Controlled Current Source/1, Product1/1, [current_left], Display1/1
  enable/1 -> AND1/1, AND/2
  Voltage Measurement2/1 -> Memory1/1
  direction/1 -> Compare To Constant/1, MATLAB Function/2(direction), Switch/2, AND1/2, Switch1/2
  [voltage_right] -> MATLAB Function/4(voltage_right)
  [voltage_left] -> MATLAB Function/3(voltage_left)
  Product/1 -> [power_right], Display3/1
  Product1/1 -> [power_left], Display4/1
  current_desired/1 -> Sum/1, Switch1/3
  [voltage_right] -> right_measurement/1
  [current_right] -> right_measurement/2
  [power_right] -> right_measurement/3
  [power_left] -> left_measurement/3
  [current_left] -> left_measurement/2
  [voltage_left] -> left_measurement/1
  right_measurement/1 -> Outport/1  "right_measurement"
  left_measurement/1 -> Outport1/1  "left_measurement"
  Voltage Measurement1/1 -> Memory/1
  Relay/1 -> AND/1
  AND/1 -> MATLAB Function/1(enable)
  Switch/1 -> Relay/1
  [voltage_left] -> Switch/3
  [voltage_right] -> Switch/1
  Memory/1 -> Product1/2, [voltage_left]
  Memory1/1 -> [voltage_right], Product/2
  Compare To Constant/1 -> AND/3
  Sum/1 -> PID Controller/1
  PID Controller/1 -> Switch1/1
  Switch1/1 -> MATLAB Function/5(current_desired)
  AND1/1 -> PID Controller/2
  Memory2/1 -> Abs/1
  MATLAB Function/2(current_right) -> [current_right], Product/1, Display2/1, Controlled Current Source1/1
  Abs/1 -> Sum/2
  connections:
  Voltage Measurement1/LConn1 -- batt_left +/RConn1 -- Controlled Current Source/RConn1
  Controlled Current Source1/RConn1 -- batt_right +/RConn1 -- Voltage Measurement2/LConn1
  Voltage Measurement2/LConn2 -- Controlled Current Source1/LConn1 -- batt_right -/RConn1
  Voltage Measurement1/LConn2 -- batt_left -/RConn1 -- Controlled Current Source/LConn1

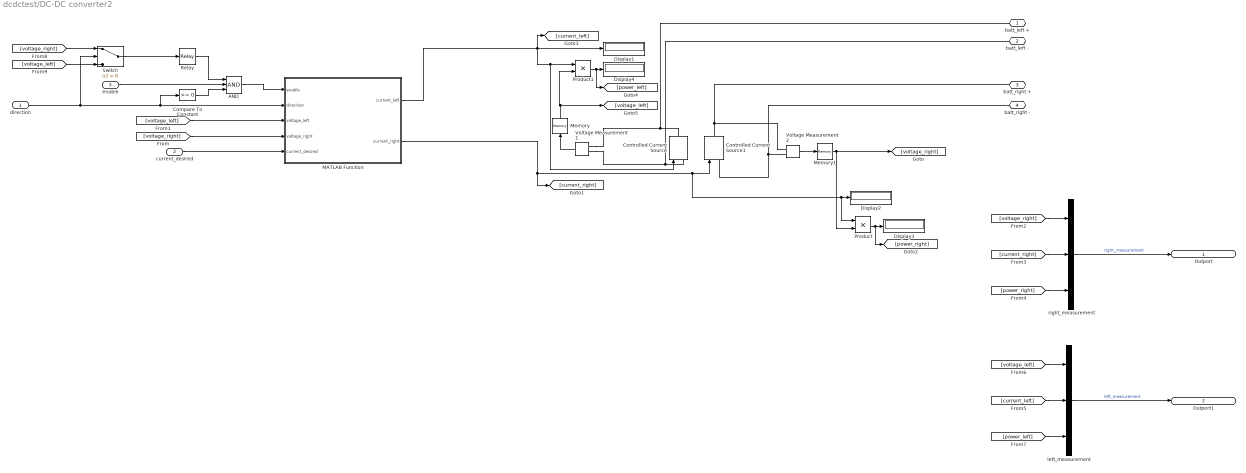
== system dcdctest/DC-DC converter2 ==
  direction : Inport
  current_desired : Inport  Port=2
  enable : Inport  Port=3
  AND : Logic  Inputs=3  IconShape=distinctive  AllPortsSameDT=off  OutDataTypeStr=boolean
  Compare To Constant : simulink/Logic and Bit Operations/Compare To Constant  relop=>=  const=0  OutDataTypeStr=boolean
  Controlled Current Source : spsControlledCurrentSourceLib/Controlled Current Source  Initialize=on  Source_Type=DC  Amplitude=0  Phase=0  Frequency=0  Measurements=None
  Controlled Current Source1 : spsControlledCurrentSourceLib/Controlled Current Source  Initialize=on  Source_Type=AC  Amplitude=0  Phase=0  Frequency=0  Measurements=None
  Display{1..4} (4 alike) : Display
  MATLAB Function : MATLAB Function  TreatAsAtomicUnit=on
  Memory : Memory
  Memory1 : Memory
  Product : Product
  Product1 : Product
  Relay : Relay  OnSwitchValue=3.5  OffSwitchValue=2
  Switch : Switch  Criteria=u2 > Threshold  SaturateOnIntegerOverflow=off  InputSameDT=off
  Voltage Measurement1 : spsVoltageMeasurementLib/Voltage Measurement  PhasorSimulation=off  OutputType=Complex  PSBequivalent=0
  Voltage Measurement2 : spsVoltageMeasurementLib/Voltage Measurement  PhasorSimulation=off  OutputType=Complex  PSBequivalent=0
  left_measurement : Mux  Inputs=3
  right_measurement : Mux  Inputs=3
  batt_left + : PMIOPort  Side=Left
  batt_left - : PMIOPort  Port=2  Side=Left
  batt_right + : PMIOPort  Port=3  Side=Right
  batt_right - : PMIOPort  Port=4  Side=Right
  Outport : Outport
  Outport1 : Outport  Port=2
  wires:
  MATLAB Function/1(current_left) -> Controlled Current Source/1, Product1/1, [current_left], Display1/1
  enable/1 -> AND/2
  Voltage Measurement2/1 -> Memory1/1
  direction/1 -> Compare To Constant/1, MATLAB Function/2(direction), Switch/2
  [voltage_right] -> MATLAB Function/4(voltage_right)
  MATLAB Function/2(current_right) -> [current_right], Product/1, Display2/1, Controlled Current Source1/1
  [voltage_left] -> MATLAB Function/3(voltage_left)
  Product/1 -> [power_right], Display3/1
  Product1/1 -> [power_left], Display4/1
  current_desired/1 -> MATLAB Function/5(current_desired)
  [voltage_right] -> right_measurement/1
  [current_right] -> right_measurement/2
  [power_right] -> right_measurement/3
  [power_left] -> left_measurement/3
  [current_left] -> left_measurement/2
  [voltage_left] -> left_measurement/1
  right_measurement/1 -> Outport/1  "right_measurement"
  left_measurement/1 -> Outport1/1  "left_measurement"
  Voltage Measurement1/1 -> Memory/1
  Relay/1 -> AND/1
  AND/1 -> MATLAB Function/1(enable)
  Switch/1 -> Relay/1
  [voltage_left] -> Switch/3
  [voltage_right] -> Switch/1
  Memory/1 -> Product1/2, [voltage_left]
  Memory1/1 -> [voltage_right], Product/2
  Compare To Constant/1 -> AND/3
  connections:
  Voltage Measurement1/LConn1 -- batt_left +/RConn1 -- Controlled Current Source/RConn1
  Controlled Current Source1/RConn1 -- batt_right +/RConn1 -- Voltage Measurement2/LConn1
  Voltage Measurement2/LConn2 -- Controlled Current Source1/LConn1 -- batt_right -/RConn1
  Voltage Measurement1/LConn2 -- batt_left -/RConn1 -- Controlled Current Source/LConn1

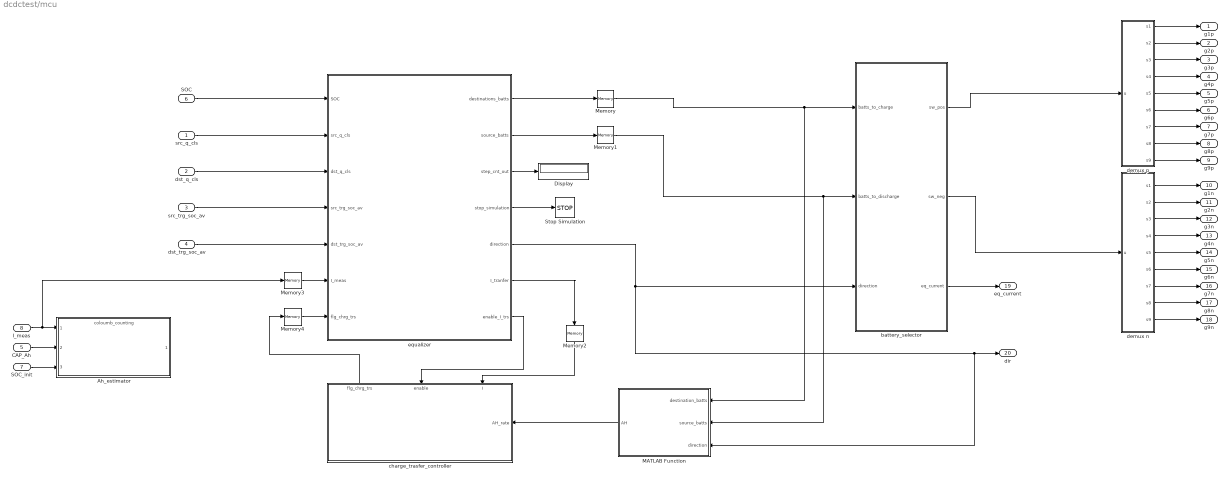
== system dcdctest/mcu ==
  src_q_cls : Inport
  dst_q_cls : Inport  Port=2
  src_trg_soc_av : Inport  Port=3
  dst_trg_soc_av : Inport  Port=4
  CAP_Ah : Inport  Port=5
  SOC : Inport  Port=6
  SOC_init : Inport  Port=7
  I_meas : Inport  Port=8
  Ah_estimator : ModelReference  ModelNameDialog=coloumb_counting.slx  SimulationMode=Normal  ModelReferenceVersion=1.13
  Display : Display
  MATLAB Function : MATLAB Function  TreatAsAtomicUnit=on
  Memory{,1..4} (5 alike) : Memory
  Stop Simulation : Stop
  battery_selector : MATLAB Function  TreatAsAtomicUnit=on
  charge_trasfer_controller : Subsystem
      settings: PortSchema="{\"entries\":[{\"content\":{\"sides\":[{\"content\":{},\"type\":\"ConnectorPlacement.EquallySpacedRectSide\",\"uuid\":\"48c70ec0-4261-4909-a719-c03e97c3e4ca\"},{\"content\":{\"connectorIds\":[\"In3\"],\"side\":\"RIGHT\"},\"type\":\"ConnectorPlacement.EquallySpacedRectSide\",\"uuid\":\"8a44a88a-c632-4005-90b8-1b0d09211c10\"},{\"content\":{\"connectorIds\":[\"Out1\",\"In1\",\"In2\"],\"side\":\"TOP\"},\"type\":\"ConnectorPlacement.EquallySpacedRectSide\",\"uuid\":\"71bafe47-820a-4a08-9919-e54bf550fba8\"}]},\"type\":\"ConnectorPlacement.EquallySpacedConnector\",\"uuid\":\"9c996bd2-099e-4131-a64b-67fbb4a72a45\"}],\"packageUris\":[\"http://schema.mathworks.com/mf0/Connector/R2020b\"],\"version\":\"1.0\"}"
  demux n : MATLAB Function  TreatAsAtomicUnit=on
  demux p : MATLAB Function  TreatAsAtomicUnit=on
  equalizer : MATLAB Function  TreatAsAtomicUnit=on
  g1p : Outport
  g2p : Outport  Port=2
  g3p : Outport  Port=3
  g4p : Outport  Port=4
  g5p : Outport  Port=5
  g6p : Outport  Port=6
  g7p : Outport  Port=7
  g8p : Outport  Port=8
  g9p : Outport  Port=9
  g1n : Outport  Port=10
  g2n : Outport  Port=11
  g3n : Outport  Port=12
  g4n : Outport  Port=13
  g5n : Outport  Port=14
  g6n : Outport  Port=15
  g7n : Outport  Port=16
  g8n : Outport  Port=17
  g9n : Outport  Port=18
  eq_current : Outport  Port=19
  dir : Outport  Port=20
  wires:
  battery_selector/3(eq_current) -> eq_current/1
  Memory/1 -> MATLAB Function/1(destination_batts), battery_selector/1(batts_to_charge)
  demux n/3(s3) -> g3n/1
  demux n/7(s7) -> g7n/1
  demux n/2(s2) -> g2n/1
  equalizer/1(destinations_batts) -> Memory/1
  dst_q_cls/1 -> equalizer/3(dst_q_cls)
  equalizer/4(stop_simulation) -> Stop Simulation/1
  demux p/7(s7) -> g7p/1
  Memory1/1 -> MATLAB Function/2(source_batts), battery_selector/2(batts_to_discharge)
  demux n/6(s6) -> g6n/1
  battery_selector/1(sw_pos) -> demux p/1(u)
  equalizer/2(source_batts) -> Memory1/1
  equalizer/3(step_cnt_out) -> Display/1
  battery_selector/2(sw_neg) -> demux n/1(u)
  src_q_cls/1 -> equalizer/2(src_q_cls)
  src_trg_soc_av/1 -> equalizer/4(src_trg_soc_av)
  demux n/5(s5) -> g5n/1
  demux n/8(s8) -> g8n/1
  dst_trg_soc_av/1 -> equalizer/5(dst_trg_soc_av)
  demux p/9(s9) -> g9p/1
  demux p/4(s4) -> g4p/1
  demux p/1(s1) -> g1p/1
  SOC/1 -> equalizer/1(SOC)
  demux p/5(s5) -> g5p/1
  demux p/2(s2) -> g2p/1
  demux p/8(s8) -> g8p/1
  demux n/1(s1) -> g1n/1
  demux n/4(s4) -> g4n/1
  demux n/9(s9) -> g9n/1
  demux p/3(s3) -> g3p/1
  demux p/6(s6) -> g6p/1
  SOC_init/1 -> Ah_estimator/3
  CAP_Ah/1 -> Ah_estimator/2
  MATLAB Function/1(AH) -> charge_trasfer_controller/3(AH_rate)
  equalizer/6(I_tranfer) -> Memory2/1
  equalizer/7(enable_I_trs) -> charge_trasfer_controller/1(enable)
  charge_trasfer_controller/1(flg_chrg_trs) -> Memory4/1
  equalizer/5(direction) -> MATLAB Function/3(direction), dir/1, battery_selector/3(direction)
  I_meas/1 -> Memory3/1, Ah_estimator/1
  Memory2/1 -> charge_trasfer_controller/2(I)
  Memory3/1 -> equalizer/6(I_meas)
  Memory4/1 -> equalizer/7(flg_chrg_trs)

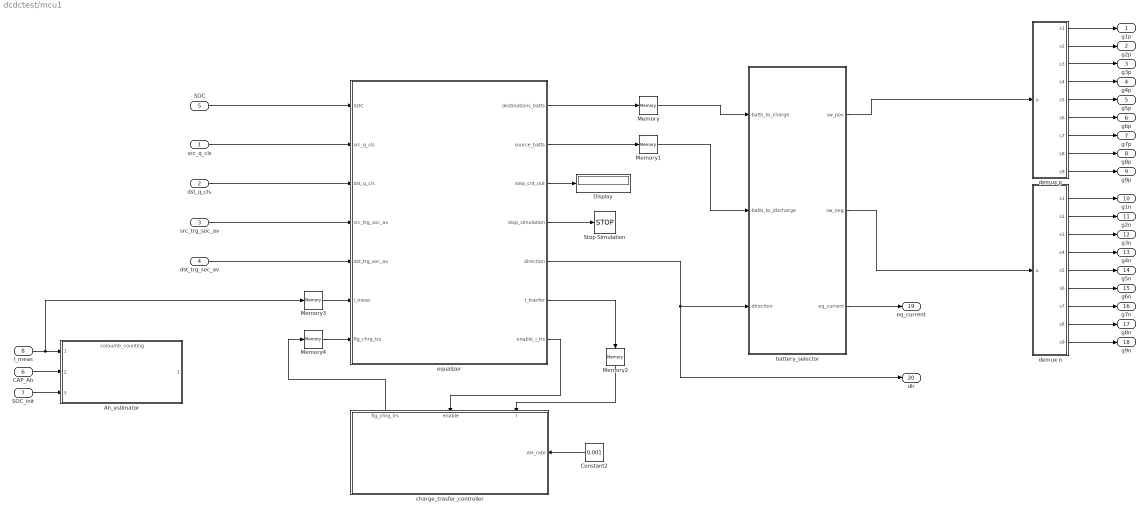
== system dcdctest/mcu1 ==
  src_q_cls : Inport
  dst_q_cls : Inport  Port=2
  src_trg_soc_av : Inport  Port=3
  dst_trg_soc_av : Inport  Port=4
  SOC : Inport  Port=5
  CAP_Ah : Inport  Port=6
  SOC_init : Inport  Port=7
  I_meas : Inport  Port=8
  Ah_estimator : ModelReference  ModelNameDialog=coloumb_counting.slx  SimulationMode=Normal  ModelReferenceVersion=1.13
  Constant2 : Constant  Value=0.001
  Display : Display
  Memory{,1..4} (5 alike) : Memory
  Stop Simulation : Stop
  battery_selector : MATLAB Function  TreatAsAtomicUnit=on
  charge_trasfer_controller : Subsystem
      settings: PortSchema="{\"entries\":[{\"content\":{\"sides\":[{\"content\":{},\"type\":\"ConnectorPlacement.EquallySpacedRectSide\",\"uuid\":\"48c70ec0-4261-4909-a719-c03e97c3e4ca\"},{\"content\":{\"connectorIds\":[\"In3\"],\"side\":\"RIGHT\"},\"type\":\"ConnectorPlacement.EquallySpacedRectSide\",\"uuid\":\"8a44a88a-c632-4005-90b8-1b0d09211c10\"},{\"content\":{\"connectorIds\":[\"Out1\",\"In1\",\"In2\"],\"side\":\"TOP\"},\"type\":\"ConnectorPlacement.EquallySpacedRectSide\",\"uuid\":\"71bafe47-820a-4a08-9919-e54bf550fba8\"}]},\"type\":\"ConnectorPlacement.EquallySpacedConnector\",\"uuid\":\"9c996bd2-099e-4131-a64b-67fbb4a72a45\"}],\"packageUris\":[\"http://schema.mathworks.com/mf0/Connector/R2020b\"],\"version\":\"1.0\"}"
  demux n : MATLAB Function  TreatAsAtomicUnit=on
  demux p : MATLAB Function  TreatAsAtomicUnit=on
  equalizer : MATLAB Function  TreatAsAtomicUnit=on
  g1p : Outport
  g2p : Outport  Port=2
  g3p : Outport  Port=3
  g4p : Outport  Port=4
  g5p : Outport  Port=5
  g6p : Outport  Port=6
  g7p : Outport  Port=7
  g8p : Outport  Port=8
  g9p : Outport  Port=9
  g1n : Outport  Port=10
  g2n : Outport  Port=11
  g3n : Outport  Port=12
  g4n : Outport  Port=13
  g5n : Outport  Port=14
  g6n : Outport  Port=15
  g7n : Outport  Port=16
  g8n : Outport  Port=17
  g9n : Outport  Port=18
  eq_current : Outport  Port=19
  dir : Outport  Port=20
  wires:
  battery_selector/3(eq_current) -> eq_current/1
  Memory/1 -> battery_selector/1(batts_to_charge)
  demux n/3(s3) -> g3n/1
  demux n/7(s7) -> g7n/1
  demux n/2(s2) -> g2n/1
  equalizer/1(destinations_batts) -> Memory/1
  dst_q_cls/1 -> equalizer/3(dst_q_cls)
  equalizer/4(stop_simulation) -> Stop Simulation/1
  demux p/7(s7) -> g7p/1
  Memory1/1 -> battery_selector/2(batts_to_discharge)
  demux n/6(s6) -> g6n/1
  battery_selector/1(sw_pos) -> demux p/1(u)
  equalizer/2(source_batts) -> Memory1/1
  equalizer/3(step_cnt_out) -> Display/1
  battery_selector/2(sw_neg) -> demux n/1(u)
  src_q_cls/1 -> equalizer/2(src_q_cls)
  src_trg_soc_av/1 -> equalizer/4(src_trg_soc_av)
  demux n/5(s5) -> g5n/1
  demux n/8(s8) -> g8n/1
  dst_trg_soc_av/1 -> equalizer/5(dst_trg_soc_av)
  demux p/9(s9) -> g9p/1
  demux p/4(s4) -> g4p/1
  demux p/1(s1) -> g1p/1
  SOC/1 -> equalizer/1(SOC)
  demux p/5(s5) -> g5p/1
  demux p/2(s2) -> g2p/1
  demux p/8(s8) -> g8p/1
  demux n/1(s1) -> g1n/1
  demux n/4(s4) -> g4n/1
  demux n/9(s9) -> g9n/1
  demux p/3(s3) -> g3p/1
  demux p/6(s6) -> g6p/1
  SOC_init/1 -> Ah_estimator/3
  CAP_Ah/1 -> Ah_estimator/2
  Constant2/1 -> charge_trasfer_controller/3(AH_rate)
  equalizer/6(I_tranfer) -> Memory2/1
  equalizer/7(enable_I_trs) -> charge_trasfer_controller/1(enable)
  charge_trasfer_controller/1(flg_chrg_trs) -> Memory4/1
  equalizer/5(direction) -> dir/1, battery_selector/3(direction)
  I_meas/1 -> Memory3/1, Ah_estimator/1
  Memory2/1 -> charge_trasfer_controller/2(I)
  Memory3/1 -> equalizer/6(I_meas)
  Memory4/1 -> equalizer/7(flg_chrg_trs)

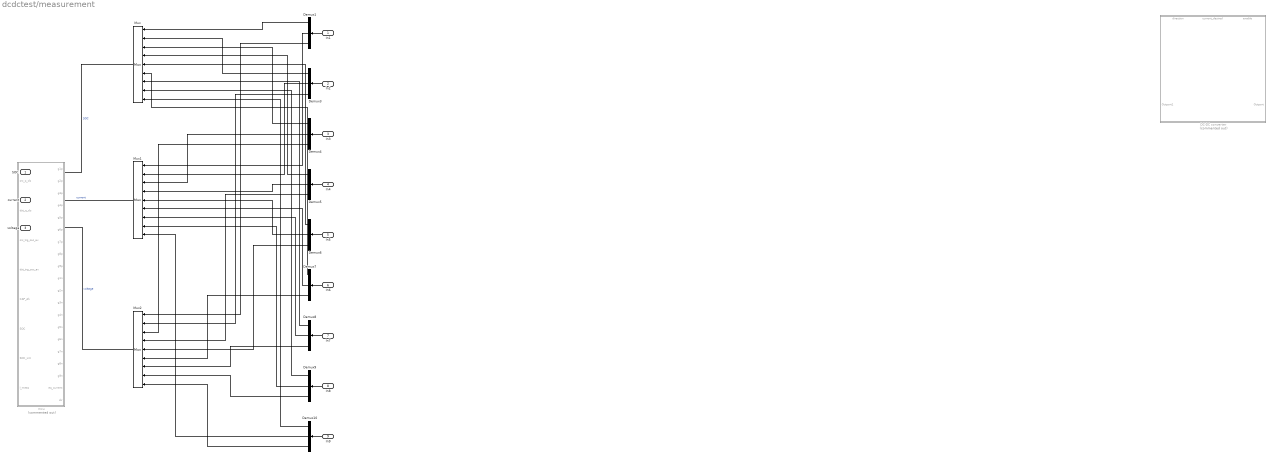
== system dcdctest/measurement ==
  In1 : Inport
  In2 : Inport  Port=2
  In3 : Inport  Port=3
  In4 : Inport  Port=4
  In5 : Inport  Port=5
  In6 : Inport  Port=6
  In7 : Inport  Port=7
  In8 : Inport  Port=8
  In9 : Inport  Port=9
  DC-DC converter : Subsystem  Commented=on
      settings: PortSchema="{\"entries\":[{\"content\":{\"sides\":[{\"content\":{\"connectorIds\":[\"LConn1\",\"LConn2\",\"Out2\"]},\"type\":\"ConnectorPlacement.EquallySpacedRectSide\",\"uuid\":\"b8e9ea21-fc6f-4abe-9815-7c96c8754cc1\"},{\"content\":{\"connectorIds\":[\"RConn1\",\"RConn2\",\"Out1\"],\"side\":\"RIGHT\"},\"type\":\"ConnectorPlacement.EquallySpacedRectSide\",\"uuid\":\"546bb611-6f28-45af-a15a-a960a3093258\"},{\"content\":{\"connectorIds\":[\"In1\",\"In2\",\"In3\"],\"side\":\"TOP\"},\"type\":\"ConnectorPlacement.EquallySpacedRectSide\",\"uuid\":\"f1a81754-76ae-41da-bcef-17d54c1fc977\"}]},\"type\":\"ConnectorPlacement.EquallySpacedConnector\",\"uuid\":\"f395fac5-4dd1-431a-bb8e-7682cfb9cc98\"}],\"packageUris\":[\"http://schema.mathworks.com/mf0/Connector/R2020b\"],\"version\":\"1.0\"}"
  Demux{1,3..10} (9 alike) : Demux  Outputs=3
  Mux : Mux  Inputs=9
  Mux1 : Mux  Inputs=9
  Mux2 : Mux  Inputs=9
  mcu : Subsystem  Commented=on
  SOC : Outport
  current : Outport  Port=2
  voltage : Outport  Port=3
  wires:
  In7/1 -> Demux8/1
  Demux6/3 -> Mux2/5
  Demux8/3 -> Mux2/7
  In5/1 -> Demux6/1
  Demux7/3 -> Mux2/6
  Demux4/1 -> Mux/3
  Demux10/3 -> Mux2/9
  Mux1/1 -> current/1  "current"
  Demux4/2 -> Mux1/3
  Demux1/3 -> Mux2/1
  Demux5/3 -> Mux2/4
  Demux10/1 -> Mux/9
  Demux4/3 -> Mux2/3
  Demux9/2 -> Mux1/8
  Demux9/3 -> Mux2/8
  Demux3/3 -> Mux2/2
  Demux9/1 -> Mux/8
  Demux10/2 -> Mux1/9
  Demux8/2 -> Mux1/7
  Demux3/1 -> Mux/2
  In6/1 -> Demux7/1
  Demux1/2 -> Mux1/1
  Demux6/1 -> Mux/5
  Demux8/1 -> Mux/7
  In1/1 -> Demux1/1
  In9/1 -> Demux10/1
  Demux7/1 -> Mux/6
  Demux1/1 -> Mux/1
  Demux3/2 -> Mux1/2
  Demux5/1 -> Mux/4
  Demux5/2 -> Mux1/4
  Demux6/2 -> Mux1/5
  Demux7/2 -> Mux1/6
  Mux/1 -> SOC/1  "SOC"
  In2/1 -> Demux3/1
  Mux2/1 -> voltage/1  "voltage"
  In3/1 -> Demux4/1
  In4/1 -> Demux5/1
  In8/1 -> Demux9/1

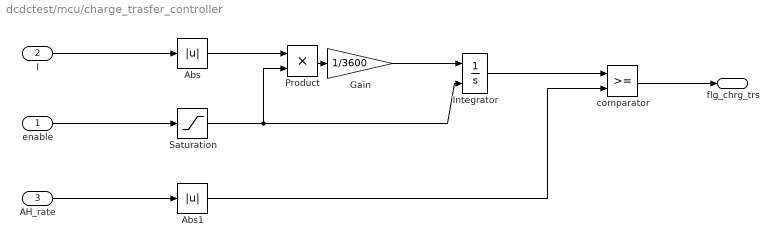
== system dcdctest/mcu/charge_trasfer_controller ==
  enable : Inport
  I : Inport  Port=2
  AH_rate : Inport  Port=3
  Abs : Abs  SaturateOnIntegerOverflow=off
  Abs1 : Abs  SaturateOnIntegerOverflow=off
  Gain : Gain  Gain=1/3600
  Integrator : Integrator  ExternalReset=either
  Product : Product
  Saturation : Saturate  UpperLimit=1  LowerLimit=0
  comparator : RelationalOperator  OutDataTypeStr=boolean  RndMeth=Simplest  InputSameDT=off
  flg_chrg_trs : Outport
  wires:
  comparator/1 -> flg_chrg_trs/1
  AH_rate/1 -> Abs1/1
  Abs/1 -> Product/1
  Integrator/1 -> comparator/1
  Product/1 -> Gain/1
  enable/1 -> Saturation/1
  Gain/1 -> Integrator/1
  Saturation/1 -> Product/2, Integrator/2
  I/1 -> Abs/1
  Abs1/1 -> comparator/2

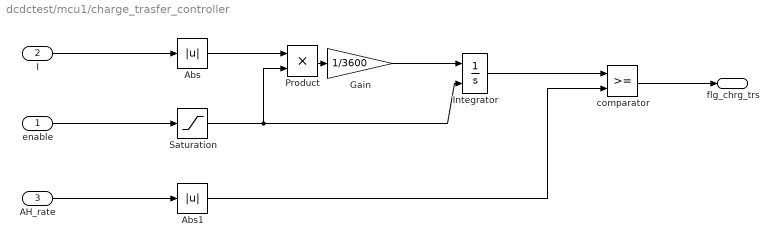
== system dcdctest/mcu1/charge_trasfer_controller ==
  enable : Inport
  I : Inport  Port=2
  AH_rate : Inport  Port=3
  Abs : Abs  SaturateOnIntegerOverflow=off
  Abs1 : Abs  SaturateOnIntegerOverflow=off
  Gain : Gain  Gain=1/3600
  Integrator : Integrator  ExternalReset=either
  Product : Product
  Saturation : Saturate  UpperLimit=1  LowerLimit=0
  comparator : RelationalOperator  OutDataTypeStr=boolean  RndMeth=Simplest  InputSameDT=off
  flg_chrg_trs : Outport
  wires:
  comparator/1 -> flg_chrg_trs/1
  AH_rate/1 -> Abs1/1
  Abs/1 -> Product/1
  Integrator/1 -> comparator/1
  Product/1 -> Gain/1
  enable/1 -> Saturation/1
  Gain/1 -> Integrator/1
  Saturation/1 -> Product/2, Integrator/2
  I/1 -> Abs/1
  Abs1/1 -> comparator/2
